simulink model "MdL_qiyi"  (Simulink 6.1)
settings: Solver=ode4  SolverMode=SingleTasking  StartTime=0.0  StopTime=5  FixedStep=0.001  RelTol=1e-3
values from neighbouring files (symbols this model uses):
  A = [0 1;8.04915 -0.09255]    [qiyi.m]
  B = [0;-8.92329]    [qiyi.m]
  C = [1 0;0 1]    [qiyi.m]
  delta_A = [0 0; 1.48068 -0.00318]*state_model    [qiyi.m]
  delta_B = [0;-0.04781]*state_model    [qiyi.m]
  K = place(A,B,P)*inv(C)    [qiyi.m]
  L = N'    [qiyi.m]
libraries: simulink x1
settings Model: LastModifiedBy=Administrator
settings DebuggingCC: SolverPrmCheckMsg=warning

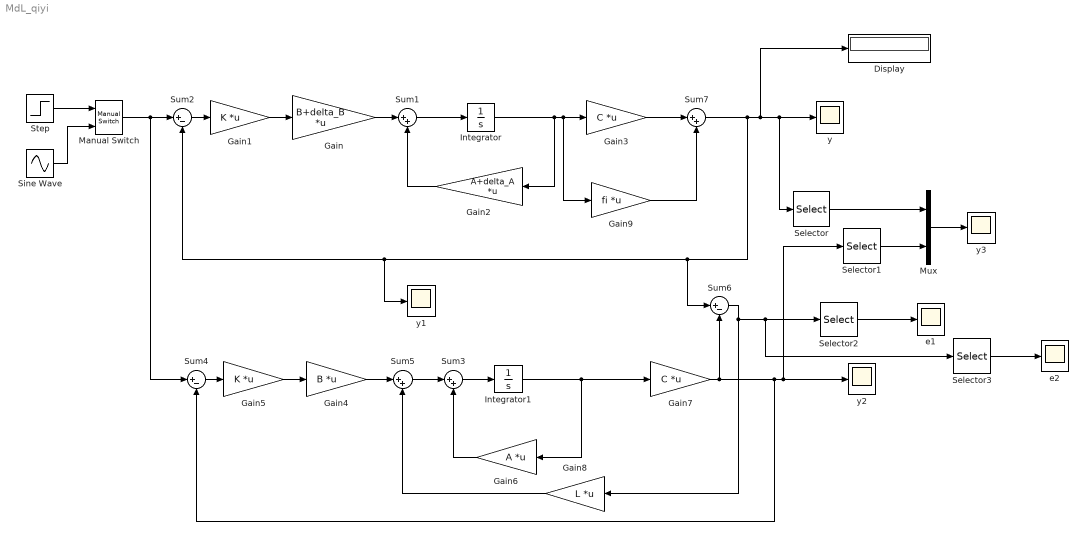
== system MdL_qiyi ==
  Display : Display
  Gain : Gain  Gain=B+delta_B  Multiplication=Matrix(K*u)
  Gain1 : Gain  Gain=K  Multiplication=Matrix(K*u)
  Gain2 : Gain  Orientation=left  Gain=A+delta_A  Multiplication=Matrix(K*u)
  Gain3 : Gain  Gain=C  Multiplication=Matrix(K*u)
  Gain4 : Gain  Gain=B  Multiplication=Matrix(K*u)
  Gain5 : Gain  Gain=K  Multiplication=Matrix(K*u)
  Gain6 : Gain  Orientation=left  Gain=A  Multiplication=Matrix(K*u)
  Gain7 : Gain  Gain=C  Multiplication=Matrix(K*u)
  Gain8 : Gain  Orientation=left  Gain=L  Multiplication=Matrix(K*u)
  Gain9 : Gain  Gain=fi  Multiplication=Matrix(K*u)
  Integrator : Integrator  InitialCondition=[2;1]
  Integrator1 : Integrator
  Manual Switch : simulink/Signal Routing/Manual Switch  sw=1  action=0
  Mux : Mux  Inputs=2
  Selector : Selector  Elements=2  InputPortWidth=2
  Selector1 : Selector  Elements=2  InputPortWidth=2
  Selector2 : Selector  InputPortWidth=2
  Selector3 : Selector  Elements=2  InputPortWidth=2
  Sine Wave : Sin  SampleTime=0
  Step : Step  Time=0  SampleTime=0
  Sum{1,3,5,7} (4 alike) : Sum  Inputs=|++
  Sum2 : Sum  Inputs=|+-
  Sum4 : Sum  Inputs=|+-
  Sum6 : Sum  Inputs=|+-
  e1 : Scope
      settings: YMin=-0.9  YMax=0  SaveName=ScopeData4
  e2 : Scope
      settings: YMin=-0.9  YMax=0  SaveName=ScopeData5
  y{,1..3} (4 alike) : Scope
      y settings: YMin=-0.9  YMax=0
      y2 settings: YMin=-0.9  YMax=0  SaveName=ScopeData2
      y3 settings: YMin=-0.9  YMax=0  SaveName=ScopeData3
  wires:
  Manual Switch/1 -> Sum2/1, Sum4/1
  Gain/1 -> Sum1/1
  Sum1/1 -> Integrator/1
  Integrator/1 -> Gain2/1, Gain3/1, Gain9/1
  Sum7/1 -> Display/1, y/1, Selector/1, Sum2/2, y1/1, Sum6/1
  Sum2/1 -> Gain1/1
  Gain1/1 -> Gain/1
  Gain4/1 -> Sum5/1
  Sum3/1 -> Integrator1/1
  Integrator1/1 -> Gain7/1, Gain6/1
  Gain6/1 -> Sum3/2
  Gain7/1 -> Sum4/2, y2/1, Selector1/1, Sum6/2
  Sum4/1 -> Gain5/1
  Gain5/1 -> Gain4/1
  Mux/1 -> y3/1
  Selector/1 -> Mux/1
  Selector1/1 -> Mux/2
  Sum5/1 -> Sum3/1
  Sum6/1 -> Gain8/1, Selector2/1, Selector3/1
  Gain8/1 -> Sum5/2
  Selector2/1 -> e1/1
  Step/1 -> Manual Switch/1
  Sine Wave/1 -> Manual Switch/2
  Gain2/1 -> Sum1/2
  Selector3/1 -> e2/1
  Gain3/1 -> Sum7/1
  Gain9/1 -> Sum7/2
